simulink model "simpleModel"  (R2018a)
settings: Solver=VariableStepAuto  StartTime=0.0  StopTime=100  RelTol=1e-3
settings Model: Creator=transmogrifier  LastModifiedBy=transmogrifier

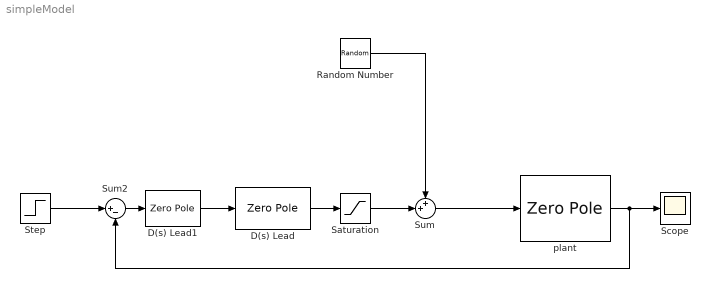
== system simpleModel ==
  D(s) Lead : ZeroPole  Zeros=[]  Poles=[-5]
  D(s) Lead1 : ZeroPole  Zeros=[-0.2668]  Poles=[-8]  Gain=[64.4]
  Random Number : RandomNumber  Variance=pi/48  SampleTime=0.1
  Saturation : Saturate  UpperLimit=pi/12  LowerLimit=-pi/12
  Scope : Scope
  Step : Step  Time=0  After=4  SampleTime=0
  Sum : Sum  Inputs=++|
  Sum2 : Sum  Inputs=|+-
  plant : ZeroPole  Zeros=[]  Poles=[0 0 -5/4]  Gain=[1.5]
  wires:
  Sum2/1 -> D(s) Lead1/1
  Step/1 -> Sum2/1
  plant/1 -> Sum2/2, Scope/1
  D(s) Lead1/1 -> D(s) Lead/1
  D(s) Lead/1 -> Saturation/1
  Random Number/1 -> Sum/1
  Saturation/1 -> Sum/2
  Sum/1 -> plant/1
